simulink library "marine_hydro"  (Simulink 7.4)
settings: Solver=ode45  SolverMode=SingleTasking  StartTime=0.0  StopTime=10.0  RelTol=1e-3
undefined symbols (not defined in the file or in its folder): Hoerner, magnitude, slcm, vessel, vesselABC
libraries: simulink x60, marine_gnc x22, marine_hydro x9
(part 4 of 4)

== system marine_hydro/Hydro Library/Wave loads (U>0)/Wave loads U = U1/psi2 ==
  k : Inport  OutDataType=sfix(16)  OutScaling=2^0
  0 or 1 : Inport  Port=2  OutDataType=sfix(16)  OutScaling=2^0
  Gain1 : Gain  Gain=20  ParameterDataType=sfix(16)  ParameterScaling=2^0  OutDataType=sfix(16)  OutScaling=2^0
  Gain2 : Gain  Gain=10  ParameterDataType=sfix(16)  ParameterScaling=2^0  OutDataType=sfix(16)  OutScaling=2^0
  Product : Product  OutDataType=sfix(16)  OutScaling=2^0  RndMeth=Zero
  Sum7 : Sum  Inputs=-+|  OutDataType=sfix(16)  OutScaling=2^0
  Sum8 : Sum  Inputs=++|  OutDataType=sfix(16)  OutScaling=2^0
  const : Constant  Value=18  OutDataType=sfix(16)  OutScaling=2^0
  psi : Outport  OutDataType=sfix(16)  OutScaling=2^0
  wires:
  0 or 1/1 -> Product/2
  Sum8/1 -> psi/1
  k/1 -> Gain2/1, Sum7/1
  Gain2/1 -> Sum8/1
  Product/1 -> Sum8/2
  Gain1/1 -> Product/1
  Sum7/1 -> Gain1/1
  const/1 -> Sum7/2

== system marine_hydro/Hydro Library/Wave loads (U>0)/Wave loads U = U2/Wave loads for heading1 ==
  eta : Inport  OutDataType=sfix(16)  OutScaling=2^0
  psi : Inport  Port=2  OutDataType=sfix(16)  OutScaling=2^0
  psi_wave : Inport  Port=3  OutDataType=sfix(16)  OutScaling=2^0
  wavenum : Inport  Port=4  OutDataType=sfix(16)  OutScaling=2^0
  Omega : Inport  Port=5  OutDataType=sfix(16)  OutScaling=2^0
  Phase : Inport  Port=6  OutDataType=sfix(16)  OutScaling=2^0
  Zeta_a : Inport  Port=7  OutDataType=sfix(16)  OutScaling=2^0
  U_idx : Inport  Port=8  OutDataType=sfix(16)  OutScaling=2^0
  Clock : Clock
      settings: Decimation=10
  Position phase : marine_gnc/Models/Environmental Loads/Utilities/Position phase  SystemSampleTime=-1
  Product1 : Product  Inputs=**  OutDataType=sfix(16)  OutScaling=2^0  SaturateOnIntegerOverflow=on  OutDataTypeStr=Inherit: Same as first input
  Sum : Sum  Inputs=-++  OutDataType=sfix(16)  OutScaling=2^0  SaturateOnIntegerOverflow=on
  Sum1 : Sum  Inputs=-+|  OutDataType=sfix(16)  OutScaling=2^0
  Wave component loop : Subsystem  TreatAsAtomicUnit=on
  Width : Width  DataType=int32
  tau_WF : Outport  OutDataType=sfix(16)  OutScaling=2^0
  tau_WD : Outport  Port=2  OutDataType=sfix(16)  OutScaling=2^0
  wires:
  psi/1 -> Sum1/1  "psi"
  U_idx/1 -> Wave component loop/6(U_idx)
  Wave component loop/2(tau_WD) -> tau_WD/1
  Sum1/1 -> Wave component loop/2(Psi_r)
  Zeta_a/1 -> Wave component loop/5(Zeta_a)
  Phase/1 -> Sum/3
  Omega/1 -> Width/1, Wave component loop/3(Omega), Product1/1
  wavenum/1 -> Position phase/2
  psi_wave/1 -> Sum1/2, Position phase/1
  eta/1 -> Position phase/3
  Wave component loop/1(tau_WF) -> tau_WF/1
  Product1/1 -> Sum/2
  Clock/1 -> Product1/2
  Sum/1 -> Wave component loop/4(Phase_tot)  "Phase_tot"
  Width/1 -> Wave component loop/1(number of  iterations)
  Position phase/1 -> Sum/1

== system marine_hydro/Hydro Library/Wave loads (U>0)/Wave loads U = U2/Wave loads for heading2 ==
  eta : Inport  OutDataType=sfix(16)  OutScaling=2^0
  psi : Inport  Port=2  OutDataType=sfix(16)  OutScaling=2^0
  psi_wave : Inport  Port=3  OutDataType=sfix(16)  OutScaling=2^0
  wavenum : Inport  Port=4  OutDataType=sfix(16)  OutScaling=2^0
  Omega : Inport  Port=5  OutDataType=sfix(16)  OutScaling=2^0
  Phase : Inport  Port=6  OutDataType=sfix(16)  OutScaling=2^0
  Zeta_a : Inport  Port=7  OutDataType=sfix(16)  OutScaling=2^0
  U : Inport  Port=8  OutDataType=sfix(16)  OutScaling=2^0
  Clock : Clock
      settings: Decimation=10
  Position phase : marine_gnc/Models/Environmental Loads/Utilities/Position phase  SystemSampleTime=-1
  Product1 : Product  Inputs=**  OutDataType=sfix(16)  OutScaling=2^0  SaturateOnIntegerOverflow=on  OutDataTypeStr=Inherit: Same as first input
  Sum : Sum  Inputs=-++  OutDataType=sfix(16)  OutScaling=2^0  SaturateOnIntegerOverflow=on
  Sum1 : Sum  Inputs=-+|  OutDataType=sfix(16)  OutScaling=2^0
  Wave component loop : Subsystem  TreatAsAtomicUnit=on
  Width : Width  DataType=int32
  tau_WF : Outport  OutDataType=sfix(16)  OutScaling=2^0
  tau_WD : Outport  Port=2  OutDataType=sfix(16)  OutScaling=2^0
  wires:
  psi/1 -> Sum1/1  "psi"
  U/1 -> Wave component loop/6(U)
  Wave component loop/2(tau_WD) -> tau_WD/1
  Sum1/1 -> Wave component loop/2(Psi_r)
  Zeta_a/1 -> Wave component loop/5(Zeta_a)
  Phase/1 -> Sum/3
  Omega/1 -> Width/1, Wave component loop/3(Omega), Product1/1
  wavenum/1 -> Position phase/2
  psi_wave/1 -> Sum1/2, Position phase/1
  eta/1 -> Position phase/3
  Wave component loop/1(tau_WF) -> tau_WF/1
  Product1/1 -> Sum/2
  Clock/1 -> Product1/2
  Sum/1 -> Wave component loop/4(Phase_tot)  "Phase_tot"
  Width/1 -> Wave component loop/1(number of  iterations)
  Position phase/1 -> Sum/1

== system marine_hydro/Hydro Library/Wave loads (U>0)/Wave loads U = U2/psi1 ==
  k : Inport  OutDataType=sfix(16)  OutScaling=2^0
  0 or 1 : Inport  Port=2  OutDataType=sfix(16)  OutScaling=2^0
  Gain1 : Gain  Gain=20  ParameterDataType=sfix(16)  ParameterScaling=2^0  OutDataType=sfix(16)  OutScaling=2^0
  Gain2 : Gain  Gain=10  ParameterDataType=sfix(16)  ParameterScaling=2^0  OutDataType=sfix(16)  OutScaling=2^0
  Product : Product  OutDataType=sfix(16)  OutScaling=2^0  RndMeth=Zero
  Sum7 : Sum  Inputs=-+|  OutDataType=sfix(16)  OutScaling=2^0
  Sum8 : Sum  Inputs=++|  OutDataType=sfix(16)  OutScaling=2^0
  const : Constant  Value=18  OutDataType=sfix(16)  OutScaling=2^0
  psi : Outport  OutDataType=sfix(16)  OutScaling=2^0
  wires:
  0 or 1/1 -> Product/2
  Sum8/1 -> psi/1
  k/1 -> Gain2/1, Sum7/1
  Gain2/1 -> Sum8/1
  Product/1 -> Sum8/2
  Gain1/1 -> Product/1
  Sum7/1 -> Gain1/1
  const/1 -> Sum7/2

== system marine_hydro/Hydro Library/Wave loads (U>0)/Wave loads U = U2/psi2 ==
  k : Inport  OutDataType=sfix(16)  OutScaling=2^0
  0 or 1 : Inport  Port=2  OutDataType=sfix(16)  OutScaling=2^0
  Gain1 : Gain  Gain=20  ParameterDataType=sfix(16)  ParameterScaling=2^0  OutDataType=sfix(16)  OutScaling=2^0
  Gain2 : Gain  Gain=10  ParameterDataType=sfix(16)  ParameterScaling=2^0  OutDataType=sfix(16)  OutScaling=2^0
  Product : Product  OutDataType=sfix(16)  OutScaling=2^0  RndMeth=Zero
  Sum7 : Sum  Inputs=-+|  OutDataType=sfix(16)  OutScaling=2^0
  Sum8 : Sum  Inputs=++|  OutDataType=sfix(16)  OutScaling=2^0
  const : Constant  Value=18  OutDataType=sfix(16)  OutScaling=2^0
  psi : Outport  OutDataType=sfix(16)  OutScaling=2^0
  wires:
  0 or 1/1 -> Product/2
  Sum8/1 -> psi/1
  k/1 -> Gain2/1, Sum7/1
  Gain2/1 -> Sum8/1
  Product/1 -> Sum8/2
  Gain1/1 -> Product/1
  Sum7/1 -> Gain1/1
  const/1 -> Sum7/2

== system marine_hydro/Hydro Library/Wave loads for heading1/Wave component loop/Force RAO tables ==
  beta : Inport  OutDataType=sfix(16)  OutScaling=2^0
  w : Inport  Port=2  OutDataType=sfix(16)  OutScaling=2^0
  U : Inport  Port=3  OutDataType=sfix(16)  OutScaling=2^0
  Lookup Table (n-D) Amp1 : simulink/Lookup Tables/Lookup Table (n-D)  numDimsPopupSelect=3  bp1=ForceRAO_Freq  bp2=vessel.headings  bp3=RAO_Vel  bp4=[1:3]  bpcell={ [1:3], [1:3] }  explicitNumDims=2  searchMode=Linear Search  cacheBpFlag=on  vectorInputFlag=off  tableData=ForceRAO_Amp{1}  interpMethod=Linear  extrapMethod=None - Clip  rangeErrorMode=Warning
  Lookup Table (n-D) Amp2 : simulink/Lookup Tables/Lookup Table (n-D)  numDimsPopupSelect=3  bp1=ForceRAO_Freq  bp2=vessel.headings  bp3=RAO_Vel  bp4=[1:3]  bpcell={ [1:3], [1:3] }  explicitNumDims=2  searchMode=Linear Search  cacheBpFlag=on  vectorInputFlag=off  tableData=ForceRAO_Amp{2}  interpMethod=Linear  extrapMethod=None - Clip  rangeErrorMode=Warning
  Lookup Table (n-D) Amp3 : simulink/Lookup Tables/Lookup Table (n-D)  numDimsPopupSelect=3  bp1=ForceRAO_Freq  bp2=vessel.headings  bp3=RAO_Vel  bp4=[1:3]  bpcell={ [1:3], [1:3] }  explicitNumDims=2  searchMode=Linear Search  cacheBpFlag=on  vectorInputFlag=off  tableData=ForceRAO_Amp{3}  interpMethod=Linear  extrapMethod=None - Clip  rangeErrorMode=Warning
  Lookup Table (n-D) Amp4 : simulink/Lookup Tables/Lookup Table (n-D)  numDimsPopupSelect=3  bp1=ForceRAO_Freq  bp2=vessel.headings  bp3=RAO_Vel  bp4=[1:3]  bpcell={ [1:3], [1:3] }  explicitNumDims=2  searchMode=Linear Search  cacheBpFlag=on  vectorInputFlag=off  tableData=ForceRAO_Amp{4}  interpMethod=Linear  extrapMethod=None - Clip  rangeErrorMode=Warning
  Lookup Table (n-D) Amp5 : simulink/Lookup Tables/Lookup Table (n-D)  numDimsPopupSelect=3  bp1=ForceRAO_Freq  bp2=vessel.headings  bp3=RAO_Vel  bp4=[1:3]  bpcell={ [1:3], [1:3] }  explicitNumDims=2  searchMode=Linear Search  cacheBpFlag=on  vectorInputFlag=off  tableData=ForceRAO_Amp{5}  interpMethod=Linear  extrapMethod=None - Clip  rangeErrorMode=Warning
  Lookup Table (n-D) Amp6 : simulink/Lookup Tables/Lookup Table (n-D)  numDimsPopupSelect=3  bp1=ForceRAO_Freq  bp2=vessel.headings  bp3=RAO_Vel  bp4=[1:3]  bpcell={ [1:3], [1:3] }  explicitNumDims=2  searchMode=Linear Search  cacheBpFlag=on  vectorInputFlag=off  tableData=ForceRAO_Amp{6}  interpMethod=Linear  extrapMethod=None - Clip  rangeErrorMode=Warning
  Lookup Table (n-D) Phase : simulink/Lookup Tables/Lookup Table (n-D)  numDimsPopupSelect=3  bp1=ForceRAO_Freq  bp2=vessel.headings  bp3=RAO_Vel  bp4=[1:3]  bpcell={ [1:3], [1:3] }  explicitNumDims=2  searchMode=Linear Search  cacheBpFlag=on  vectorInputFlag=off  tableData=ForceRAO_Phase{3}  interpMethod=Linear  extrapMethod=None - Clip  rangeErrorMode=Warning
  Lookup Table (n-D) Phase1 : simulink/Lookup Tables/Lookup Table (n-D)  numDimsPopupSelect=3  bp1=ForceRAO_Freq  bp2=vessel.headings  bp3=RAO_Vel  bp4=[1:3]  bpcell={ [1:3], [1:3] }  explicitNumDims=2  searchMode=Linear Search  cacheBpFlag=on  vectorInputFlag=off  tableData=ForceRAO_Phase{1}  interpMethod=Linear  extrapMethod=None - Clip  rangeErrorMode=Warning
  Lookup Table (n-D) Phase2 : simulink/Lookup Tables/Lookup Table (n-D)  numDimsPopupSelect=3  bp1=ForceRAO_Freq  bp2=vessel.headings  bp3=RAO_Vel  bp4=[1:3]  bpcell={ [1:3], [1:3] }  explicitNumDims=2  searchMode=Linear Search  cacheBpFlag=on  vectorInputFlag=off  tableData=ForceRAO_Phase{2}  interpMethod=Linear  extrapMethod=None - Clip  rangeErrorMode=Warning
  Lookup Table (n-D) Phase4 : simulink/Lookup Tables/Lookup Table (n-D)  numDimsPopupSelect=3  bp1=ForceRAO_Freq  bp2=vessel.headings  bp3=RAO_Vel  bp4=[1:3]  bpcell={ [1:3], [1:3] }  explicitNumDims=2  searchMode=Linear Search  cacheBpFlag=on  vectorInputFlag=off  tableData=ForceRAO_Phase{4}  interpMethod=Linear  extrapMethod=None - Clip  rangeErrorMode=Warning
  Lookup Table (n-D) Phase5 : simulink/Lookup Tables/Lookup Table (n-D)  numDimsPopupSelect=3  bp1=ForceRAO_Freq  bp2=vessel.headings  bp3=RAO_Vel  bp4=[1:3]  bpcell={ [1:3], [1:3] }  explicitNumDims=2  searchMode=Linear Search  cacheBpFlag=on  vectorInputFlag=off  tableData=ForceRAO_Phase{5}  interpMethod=Linear  extrapMethod=None - Clip  rangeErrorMode=Warning
  Lookup Table (n-D) Phase6 : simulink/Lookup Tables/Lookup Table (n-D)  numDimsPopupSelect=3  bp1=ForceRAO_Freq  bp2=vessel.headings  bp3=RAO_Vel  bp4=[1:3]  bpcell={ [1:3], [1:3] }  explicitNumDims=2  searchMode=Linear Search  cacheBpFlag=on  vectorInputFlag=off  tableData=ForceRAO_Phase{6}  interpMethod=Linear  extrapMethod=None - Clip  rangeErrorMode=Warning
  Mux1 : Mux  Inputs=6
  Mux2 : Mux  Inputs=6
  amp : Outport  OutDataType=sfix(16)  OutScaling=2^0
  phase : Outport  Port=2  OutDataType=sfix(16)  OutScaling=2^0
  wires:
  Mux1/1 -> amp/1
  Mux2/1 -> phase/1
  Lookup Table (n-D) Amp6/1 -> Mux1/6
  Lookup Table (n-D) Amp2/1 -> Mux1/2
  Lookup Table (n-D) Amp5/1 -> Mux1/5
  Lookup Table (n-D) Amp3/1 -> Mux1/3
  Lookup Table (n-D) Amp1/1 -> Mux1/1
  U/1 -> Lookup Table (n-D) Phase5/3, Lookup Table (n-D) Phase6/3, Lookup Table (n-D) Phase4/3, Lookup Table (n-D) Phase/3, Lookup Table (n-D) Phase2/3, Lookup Table (n-D) Phase1/3, Lookup Table (n-D) Amp6/3, Lookup Table (n-D) Amp5/3, Lookup Table (n-D) Amp4/3, Lookup Table (n-D) Amp3/3, Lookup Table (n-D) Amp2/3, Lookup Table (n-D) Amp1/3
  Lookup Table (n-D) Amp4/1 -> Mux1/4
  Lookup Table (n-D) Phase6/1 -> Mux2/6
  Lookup Table (n-D) Phase2/1 -> Mux2/2
  Lookup Table (n-D) Phase4/1 -> Mux2/4
  beta/1 -> Lookup Table (n-D) Phase5/2, Lookup Table (n-D) Phase6/2, Lookup Table (n-D) Phase4/2, Lookup Table (n-D) Phase/2, Lookup Table (n-D) Phase2/2, Lookup Table (n-D) Phase1/2, Lookup Table (n-D) Amp6/2, Lookup Table (n-D) Amp5/2, Lookup Table (n-D) Amp4/2, Lookup Table (n-D) Amp3/2, Lookup Table (n-D) Amp2/2, Lookup Table (n-D) Amp1/2
  Lookup Table (n-D) Phase1/1 -> Mux2/1
  Lookup Table (n-D) Phase/1 -> Mux2/3
  Lookup Table (n-D) Phase5/1 -> Mux2/5
  w/1 -> Lookup Table (n-D) Phase5/1, Lookup Table (n-D) Phase6/1, Lookup Table (n-D) Phase4/1, Lookup Table (n-D) Phase/1, Lookup Table (n-D) Phase2/1, Lookup Table (n-D) Phase1/1, Lookup Table (n-D) Amp6/1, Lookup Table (n-D) Amp5/1, Lookup Table (n-D) Amp4/1, Lookup Table (n-D) Amp3/1, Lookup Table (n-D) Amp2/1, Lookup Table (n-D) Amp1/1

== system marine_hydro/Hydro Library/Wave loads for heading1/Wave component loop/WD RAO tables ==
  beta : Inport  OutDataType=sfix(16)  OutScaling=2^0
  w : Inport  Port=2  OutDataType=sfix(16)  OutScaling=2^0
  U : Inport  Port=3  OutDataType=sfix(16)  OutScaling=2^0
  Constant : Constant  Value=0  OutDataType=sfix(16)  OutScaling=2^0
  Lookup Table (n-D)  Wavedrift 1 : simulink/Lookup Tables/Lookup Table (n-D)  numDimsPopupSelect=3  bp1=WD_Freq  bp2=vessel.headings  bp3=RAO_Vel  bp4=[1:3]  bpcell={ [1:3], [1:3] }  explicitNumDims=2  searchMode=Linear Search  cacheBpFlag=on  vectorInputFlag=off  tableData=WD_Amp{1}  interpMethod=Linear  extrapMethod=None - Clip  rangeErrorMode=Warning
  Lookup Table (n-D)  Wavedrift 2 : simulink/Lookup Tables/Lookup Table (n-D)  numDimsPopupSelect=3  bp1=WD_Freq  bp2=vessel.headings  bp3=RAO_Vel  bp4=[1:3]  bpcell={ [1:3], [1:3] }  explicitNumDims=2  searchMode=Linear Search  cacheBpFlag=on  vectorInputFlag=off  tableData=WD_Amp{2}  interpMethod=Linear  extrapMethod=None - Clip  rangeErrorMode=Warning
  Lookup Table (n-D)  Wavedrift 3 : simulink/Lookup Tables/Lookup Table (n-D)  numDimsPopupSelect=3  bp1=WD_Freq  bp2=vessel.headings  bp3=RAO_Vel  bp4=[1:3]  bpcell={ [1:3], [1:3] }  explicitNumDims=2  searchMode=Linear Search  cacheBpFlag=on  vectorInputFlag=off  tableData=WD_Amp{3}  interpMethod=Linear  extrapMethod=None - Clip  rangeErrorMode=Warning
  Mux1 : Mux  Inputs=6
  amp : Outport  OutDataType=sfix(16)  OutScaling=2^0
  wires:
  Mux1/1 -> amp/1
  Lookup Table (n-D)  Wavedrift 3/1 -> Mux1/6
  Lookup Table (n-D)  Wavedrift 2/1 -> Mux1/2
  Lookup Table (n-D)  Wavedrift 1/1 -> Mux1/1
  U/1 -> Lookup Table (n-D)  Wavedrift 2/3, Lookup Table (n-D)  Wavedrift 3/3, Lookup Table (n-D)  Wavedrift 1/3
  beta/1 -> Lookup Table (n-D)  Wavedrift 2/2, Lookup Table (n-D)  Wavedrift 3/2, Lookup Table (n-D)  Wavedrift 1/2
  Constant/1 -> Mux1/3, Mux1/4, Mux1/5
  w/1 -> Lookup Table (n-D)  Wavedrift 2/1, Lookup Table (n-D)  Wavedrift 3/1, Lookup Table (n-D)  Wavedrift 1/1

== system marine_hydro/Hydro Library/Wave loads for heading1/Wave component loop/[-pi pi] to [0 2pi] ==
  note: x
  x [-pi pi] : Inport  OutDataType=sfix(16)  OutScaling=2^0
  Constant : Constant  Value=2*pi  OutDataType=sfix(16)  OutScaling=2^0
  Constant1 : Constant  Value=0  OutDataType=sfix(16)  OutScaling=2^0
  Sign : Signum
  Sum : Sum  Inputs=|++  OutDataType=sfix(16)  OutScaling=2^0  SaturateOnIntegerOverflow=on
  Switch : Switch
  0<y<2pi : Outport  OutDataType=sfix(16)  OutScaling=2^0
  wires:
  x [-pi pi]/1 -> Sign/1, Sum/2
  Switch/1 -> Sum/1
  Sum/1 -> 0<y<2pi/1
  Sign/1 -> Switch/2
  Constant/1 -> Switch/3
  Constant1/1 -> Switch/1

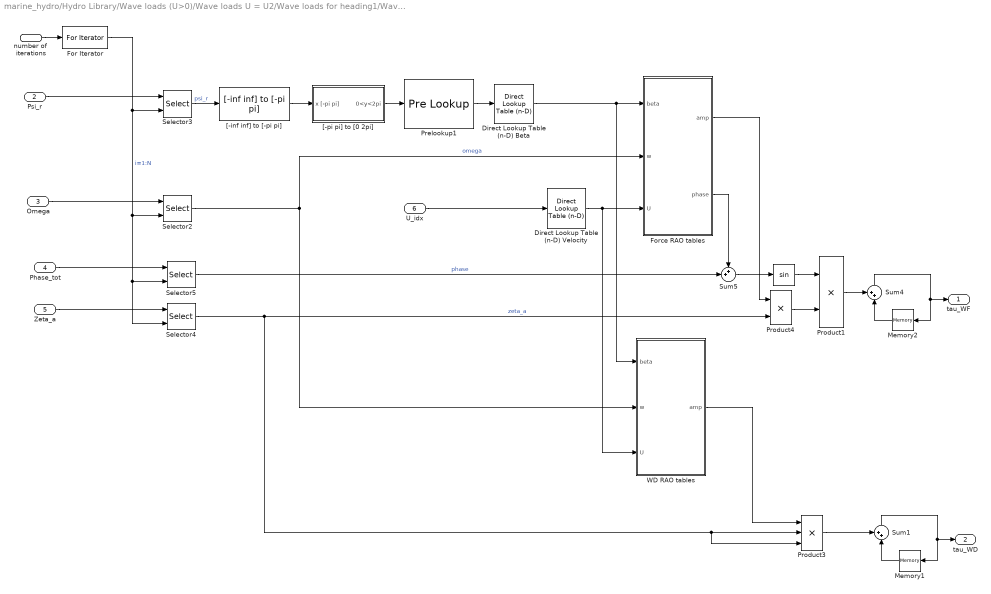
== system marine_hydro/Hydro Library/Wave loads (U>0)/Wave loads U = U2/Wave loads for heading1/Wave component loop ==
  number of  iterations : Inport  OutDataType=sfix(16)  OutScaling=2^0
  Psi_r : Inport  Port=2  OutDataType=sfix(16)  OutScaling=2^0
  Omega : Inport  Port=3  OutDataType=sfix(16)  OutScaling=2^0
  Phase_tot : Inport  Port=4  OutDataType=sfix(16)  OutScaling=2^0
  Zeta_a : Inport  Port=5  OutDataType=sfix(16)  OutScaling=2^0
  U_idx : Inport  Port=6  OutDataType=sfix(16)  OutScaling=2^0
  "                " : Trigonometry
  Direct Lookup Table (n-D) Beta : simulink/Lookup Tables/Direct Lookup Table (n-D)  maskTabDims=1  explicitNumDims=1  outDims=Element  tabIsInput=off  mxTable=vessel.headings  clipFlag=Warning  samptime=-1
  Direct Lookup Table (n-D) Velocity : simulink/Lookup Tables/Direct Lookup Table (n-D)  maskTabDims=1  explicitNumDims=1  outDims=Element  tabIsInput=off  mxTable=RAO_Vel  clipFlag=Warning  samptime=-1
  For Iterator : ForIterator  ResetStates=reset  IterationSource=external  IterationVariableDataType=double
  Force RAO tables : Subsystem  AncestorBlock=marine_gnc/Models/Environmental Loads/Utilities/RAO tables
      mask Type: RAO table lookup
      mask Description:
      | Perform 3D table lookup in 6DOF RAO amplitudes and phases, using the relative wave heading psi_r, wave frequency omega and vessel velocity vel as inputs. See documentation of the Motion RAO block or Force RAO block for details. A warning is issued if the input is outside the range spanned by the RAOs.
      | 
      | Author: Oyvind N. Smogeli and Thor I. Fossen, 2005-05-03
  Memory1 : Memory  X0=[0 0 0 0 0 0]'  InheritSampleTime=on
  Memory2 : Memory  X0=[0 0 0 0 0 0]'  InheritSampleTime=on
  Prelookup1 : PreLookup  BreakpointsData=vessel.headings  IndexSearchMethod=Evenly spaced points  BeginIndexSearchUsingPreviousIndexResult=on  OutputOnlyTheIndex=on  IndexDataType=sfix(16)  FractionDataType=sfix(16)  FractionScaling=2^0
  Product1 : Product  OutDataType=sfix(16)  OutScaling=2^0  SaturateOnIntegerOverflow=on  OutDataTypeStr=Inherit: Same as first input
  Product3 : Product  Inputs=3  OutDataType=sfix(16)  OutScaling=2^0  SaturateOnIntegerOverflow=on  OutDataTypeStr=Inherit: Same as first input
  Product4 : Product  OutDataType=sfix(16)  OutScaling=2^0  SaturateOnIntegerOverflow=on  OutDataTypeStr=Inherit: Same as first input
  Selector{2..5} (4 alike) : Selector  IndexOptions=Index vector (port)  Indices=[1 3]  OutputSizes=1
  Sum1 : Sum  Inputs=++|  OutDataType=sfix(16)  OutScaling=2^0  SaturateOnIntegerOverflow=on
  Sum4 : Sum  Inputs=++|  OutDataType=sfix(16)  OutScaling=2^0  SaturateOnIntegerOverflow=on
  Sum5 : Sum  Inputs=++|  OutDataType=sfix(16)  OutScaling=2^0  SaturateOnIntegerOverflow=on
  WD RAO tables : Subsystem  AncestorBlock=marine_gnc/Models/Environmental Loads/Utilities/RAO tables
      mask Type: RAO table lookup
      mask Description:
      | Perform 3D table lookup in 6DOF RAO amplitudes and phases, using the relative wave heading psi_r, wave frequency omega and vessel velocity vel as inputs. See documentation of the Motion RAO block or Force RAO block for details. A warning is issued if the input is outside the range spanned by the RAOs.
      | 
      | Author: Oyvind N. Smogeli and Thor I. Fossen, 2005-05-03
  "[-inf inf] to [-pi pi]" : marine_gnc/Utilities/Math Operations/[-inf inf] to [-pi pi]  SystemSampleTime=-1
  "[-pi pi] to [0 2pi]" : Subsystem
      mask Type: [-inf inf] to [-pi pi]
      mask Description: Converts an angle in rad to (-pi pi)
  tau_WF : Outport  OutDataType=sfix(16)  OutScaling=2^0
  tau_WD : Outport  Port=2  OutDataType=sfix(16)  OutScaling=2^0
  wires:
  Direct Lookup Table (n-D) Velocity/1 -> WD RAO tables/3(U), Force RAO tables/3(U)
  U_idx/1 -> Direct Lookup Table (n-D) Velocity/1
  Direct Lookup Table (n-D) Beta/1 -> WD RAO tables/1(beta), Force RAO tables/1(beta)
  Prelookup1/1 -> Direct Lookup Table (n-D) Beta/1
  "[-inf inf] to [-pi pi]"/1 -> "[-pi pi] to [0 2pi]"/1(x [-pi pi])
  For Iterator/1 -> Selector5/2, Selector4/2, Selector2/2, Selector3/2  "i=1:N"
  Selector2/1 -> WD RAO tables/2(w), Force RAO tables/2(w)  "omega"
  "[-pi pi] to [0 2pi]"/1(0<y<2pi) -> Prelookup1/1
  WD RAO tables/1(amp) -> Product3/1
  Product3/1 -> Sum1/1
  Memory1/1 -> Sum1/2
  Sum1/1 -> tau_WD/1, Memory1/1
  Product4/1 -> Product1/2
  "                "/1 -> Product1/1
  Selector3/1 -> "[-inf inf] to [-pi pi]"/1  "psi_r"
  Selector5/1 -> Sum5/2  "phase"
  Product1/1 -> Sum4/1
  Memory2/1 -> Sum4/2
  Sum4/1 -> tau_WF/1, Memory2/1
  number of  iterations/1 -> For Iterator/1
  Omega/1 -> Selector2/1
  Psi_r/1 -> Selector3/1
  Force RAO tables/1(amp) -> Product4/1
  Force RAO tables/2(phase) -> Sum5/1
  Phase_tot/1 -> Selector5/1
  Zeta_a/1 -> Selector4/1
  Sum5/1 -> "                "/1
  Selector4/1 -> Product3/3, Product3/2, Product4/2  "zeta_a"

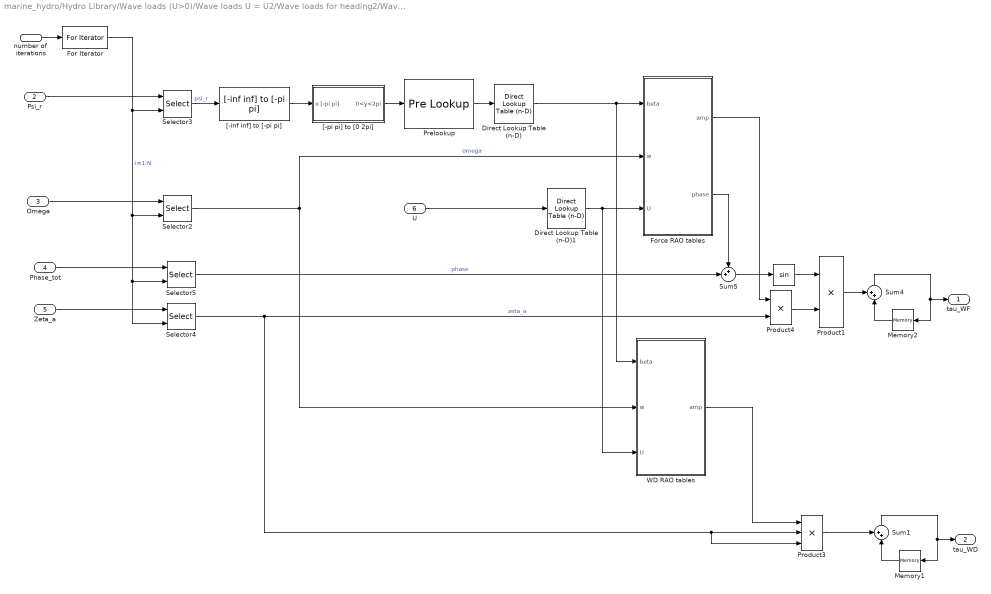
== system marine_hydro/Hydro Library/Wave loads (U>0)/Wave loads U = U2/Wave loads for heading2/Wave component loop ==
  number of  iterations : Inport  OutDataType=sfix(16)  OutScaling=2^0
  Psi_r : Inport  Port=2  OutDataType=sfix(16)  OutScaling=2^0
  Omega : Inport  Port=3  OutDataType=sfix(16)  OutScaling=2^0
  Phase_tot : Inport  Port=4  OutDataType=sfix(16)  OutScaling=2^0
  Zeta_a : Inport  Port=5  OutDataType=sfix(16)  OutScaling=2^0
  U : Inport  Port=6  OutDataType=sfix(16)  OutScaling=2^0
  "                " : Trigonometry
  Direct Lookup Table (n-D) : simulink/Lookup Tables/Direct Lookup Table (n-D)  maskTabDims=1  explicitNumDims=1  outDims=Element  tabIsInput=off  mxTable=vessel.headings  clipFlag=Warning  samptime=-1
  Direct Lookup Table (n-D)1 : simulink/Lookup Tables/Direct Lookup Table (n-D)  maskTabDims=1  explicitNumDims=1  outDims=Element  tabIsInput=off  mxTable=RAO_Vel  clipFlag=Warning  samptime=-1
  For Iterator : ForIterator  ResetStates=reset  IterationSource=external  IterationVariableDataType=double
  Force RAO tables : Subsystem  AncestorBlock=marine_gnc/Models/Environmental Loads/Utilities/RAO tables
      mask Type: RAO table lookup
      mask Description:
      | Perform 3D table lookup in 6DOF RAO amplitudes and phases, using the relative wave heading psi_r, wave frequency omega and vessel velocity vel as inputs. See documentation of the Motion RAO block or Force RAO block for details. A warning is issued if the input is outside the range spanned by the RAOs.
      | 
      | Copyright (C) NTNU 2005
      | 
      | Author: Oyvind N. Smogeli, 2005-05-03
  Memory1 : Memory  X0=[0 0 0 0 0 0]'  InheritSampleTime=on
  Memory2 : Memory  X0=[0 0 0 0 0 0]'  InheritSampleTime=on
  Prelookup : PreLookup  BreakpointsData=vessel.headings  IndexSearchMethod=Evenly spaced points  BeginIndexSearchUsingPreviousIndexResult=on  OutputOnlyTheIndex=on  IndexDataType=sfix(16)  FractionDataType=sfix(16)  FractionScaling=2^0
  Product1 : Product  OutDataType=sfix(16)  OutScaling=2^0  SaturateOnIntegerOverflow=on  OutDataTypeStr=Inherit: Same as first input
  Product3 : Product  Inputs=3  OutDataType=sfix(16)  OutScaling=2^0  SaturateOnIntegerOverflow=on  OutDataTypeStr=Inherit: Same as first input
  Product4 : Product  OutDataType=sfix(16)  OutScaling=2^0  SaturateOnIntegerOverflow=on  OutDataTypeStr=Inherit: Same as first input
  Selector{2..5} (4 alike) : Selector  IndexOptions=Index vector (port)  Indices=[1 3]  OutputSizes=1
  Sum1 : Sum  Inputs=++|  OutDataType=sfix(16)  OutScaling=2^0  SaturateOnIntegerOverflow=on
  Sum4 : Sum  Inputs=++|  OutDataType=sfix(16)  OutScaling=2^0  SaturateOnIntegerOverflow=on
  Sum5 : Sum  Inputs=++|  OutDataType=sfix(16)  OutScaling=2^0  SaturateOnIntegerOverflow=on
  WD RAO tables : Subsystem  AncestorBlock=marine_gnc/Models/Environmental Loads/Utilities/RAO tables
      mask Type: RAO table lookup
      mask Description:
      | Perform 3D table lookup in 6DOF RAO amplitudes and phases, using the relative wave heading psi_r, wave frequency omega and vessel velocity vel as inputs. See documentation of the Motion RAO block or Force RAO block for details. A warning is issued if the input is outside the range spanned by the RAOs.
      | 
      | Copyright (C) NTNU 2005
      | 
      | Author: Oyvind N. Smogeli, 2005-05-03
  "[-inf inf] to [-pi pi]" : marine_gnc/Utilities/Math Operations/[-inf inf] to [-pi pi]  SystemSampleTime=-1
  "[-pi pi] to [0 2pi]" : Subsystem
      mask Type: [-inf inf] to [-pi pi]
      mask Description: Converts an angle in rad to (-pi pi)
  tau_WF : Outport  OutDataType=sfix(16)  OutScaling=2^0
  tau_WD : Outport  Port=2  OutDataType=sfix(16)  OutScaling=2^0
  wires:
  Direct Lookup Table (n-D)1/1 -> WD RAO tables/3(U), Force RAO tables/3(U)
  Direct Lookup Table (n-D)/1 -> WD RAO tables/1(beta), Force RAO tables/1(beta)
  Prelookup/1 -> Direct Lookup Table (n-D)/1
  "[-inf inf] to [-pi pi]"/1 -> "[-pi pi] to [0 2pi]"/1(x [-pi pi])
  For Iterator/1 -> Selector5/2, Selector4/2, Selector2/2, Selector3/2  "i=1:N"
  Selector2/1 -> WD RAO tables/2(w), Force RAO tables/2(w)  "omega"
  "[-pi pi] to [0 2pi]"/1(0<y<2pi) -> Prelookup/1
  WD RAO tables/1(amp) -> Product3/1
  Product3/1 -> Sum1/1
  Memory1/1 -> Sum1/2
  Sum1/1 -> tau_WD/1, Memory1/1
  Product4/1 -> Product1/2
  "                "/1 -> Product1/1
  Selector3/1 -> "[-inf inf] to [-pi pi]"/1  "psi_r"
  Selector5/1 -> Sum5/2  "phase"
  Product1/1 -> Sum4/1
  Memory2/1 -> Sum4/2
  Sum4/1 -> tau_WF/1, Memory2/1
  number of  iterations/1 -> For Iterator/1
  Omega/1 -> Selector2/1
  Psi_r/1 -> Selector3/1
  U/1 -> Direct Lookup Table (n-D)1/1
  Force RAO tables/1(amp) -> Product4/1
  Force RAO tables/2(phase) -> Sum5/1
  Phase_tot/1 -> Selector5/1
  Zeta_a/1 -> Selector4/1
  Sum5/1 -> "                "/1
  Selector4/1 -> Product3/3, Product3/2, Product4/2  "zeta_a"

== system marine_hydro/Hydro Library/Wave loads (U>0)/Wave loads U = U2/Wave loads for heading1/Wave component loop/Force RAO tables ==
  beta : Inport  OutDataType=sfix(16)  OutScaling=2^0
  w : Inport  Port=2  OutDataType=sfix(16)  OutScaling=2^0
  U : Inport  Port=3  OutDataType=sfix(16)  OutScaling=2^0
  Lookup Table (n-D) Amp1 : simulink/Lookup Tables/Lookup Table (n-D)  numDimsPopupSelect=3  bp1=ForceRAO_Freq  bp2=vessel.headings  bp3=RAO_Vel  bp4=[1:3]  bpcell={ [1:3], [1:3] }  explicitNumDims=2  searchMode=Linear Search  cacheBpFlag=on  vectorInputFlag=off  tableData=ForceRAO_Amp{1}  interpMethod=Linear  extrapMethod=None - Clip  rangeErrorMode=Warning
  Lookup Table (n-D) Amp2 : simulink/Lookup Tables/Lookup Table (n-D)  numDimsPopupSelect=3  bp1=ForceRAO_Freq  bp2=vessel.headings  bp3=RAO_Vel  bp4=[1:3]  bpcell={ [1:3], [1:3] }  explicitNumDims=2  searchMode=Linear Search  cacheBpFlag=on  vectorInputFlag=off  tableData=ForceRAO_Amp{2}  interpMethod=Linear  extrapMethod=None - Clip  rangeErrorMode=Warning
  Lookup Table (n-D) Amp3 : simulink/Lookup Tables/Lookup Table (n-D)  numDimsPopupSelect=3  bp1=ForceRAO_Freq  bp2=vessel.headings  bp3=RAO_Vel  bp4=[1:3]  bpcell={ [1:3], [1:3] }  explicitNumDims=2  searchMode=Linear Search  cacheBpFlag=on  vectorInputFlag=off  tableData=ForceRAO_Amp{3}  interpMethod=Linear  extrapMethod=None - Clip  rangeErrorMode=Warning
  Lookup Table (n-D) Amp4 : simulink/Lookup Tables/Lookup Table (n-D)  numDimsPopupSelect=3  bp1=ForceRAO_Freq  bp2=vessel.headings  bp3=RAO_Vel  bp4=[1:3]  bpcell={ [1:3], [1:3] }  explicitNumDims=2  searchMode=Linear Search  cacheBpFlag=on  vectorInputFlag=off  tableData=ForceRAO_Amp{4}  interpMethod=Linear  extrapMethod=None - Clip  rangeErrorMode=Warning
  Lookup Table (n-D) Amp5 : simulink/Lookup Tables/Lookup Table (n-D)  numDimsPopupSelect=3  bp1=ForceRAO_Freq  bp2=vessel.headings  bp3=RAO_Vel  bp4=[1:3]  bpcell={ [1:3], [1:3] }  explicitNumDims=2  searchMode=Linear Search  cacheBpFlag=on  vectorInputFlag=off  tableData=ForceRAO_Amp{5}  interpMethod=Linear  extrapMethod=None - Clip  rangeErrorMode=Warning
  Lookup Table (n-D) Amp6 : simulink/Lookup Tables/Lookup Table (n-D)  numDimsPopupSelect=3  bp1=ForceRAO_Freq  bp2=vessel.headings  bp3=RAO_Vel  bp4=[1:3]  bpcell={ [1:3], [1:3] }  explicitNumDims=2  searchMode=Linear Search  cacheBpFlag=on  vectorInputFlag=off  tableData=ForceRAO_Amp{6}  interpMethod=Linear  extrapMethod=None - Clip  rangeErrorMode=Warning
  Lookup Table (n-D) Phase : simulink/Lookup Tables/Lookup Table (n-D)  numDimsPopupSelect=3  bp1=ForceRAO_Freq  bp2=vessel.headings  bp3=RAO_Vel  bp4=[1:3]  bpcell={ [1:3], [1:3] }  explicitNumDims=2  searchMode=Linear Search  cacheBpFlag=on  vectorInputFlag=off  tableData=ForceRAO_Phase{3}  interpMethod=Linear  extrapMethod=None - Clip  rangeErrorMode=Warning
  Lookup Table (n-D) Phase1 : simulink/Lookup Tables/Lookup Table (n-D)  numDimsPopupSelect=3  bp1=ForceRAO_Freq  bp2=vessel.headings  bp3=RAO_Vel  bp4=[1:3]  bpcell={ [1:3], [1:3] }  explicitNumDims=2  searchMode=Linear Search  cacheBpFlag=on  vectorInputFlag=off  tableData=ForceRAO_Phase{1}  interpMethod=Linear  extrapMethod=None - Clip  rangeErrorMode=Warning
  Lookup Table (n-D) Phase2 : simulink/Lookup Tables/Lookup Table (n-D)  numDimsPopupSelect=3  bp1=ForceRAO_Freq  bp2=vessel.headings  bp3=RAO_Vel  bp4=[1:3]  bpcell={ [1:3], [1:3] }  explicitNumDims=2  searchMode=Linear Search  cacheBpFlag=on  vectorInputFlag=off  tableData=ForceRAO_Phase{2}  interpMethod=Linear  extrapMethod=None - Clip  rangeErrorMode=Warning
  Lookup Table (n-D) Phase4 : simulink/Lookup Tables/Lookup Table (n-D)  numDimsPopupSelect=3  bp1=ForceRAO_Freq  bp2=vessel.headings  bp3=RAO_Vel  bp4=[1:3]  bpcell={ [1:3], [1:3] }  explicitNumDims=2  searchMode=Linear Search  cacheBpFlag=on  vectorInputFlag=off  tableData=ForceRAO_Phase{4}  interpMethod=Linear  extrapMethod=None - Clip  rangeErrorMode=Warning
  Lookup Table (n-D) Phase5 : simulink/Lookup Tables/Lookup Table (n-D)  numDimsPopupSelect=3  bp1=ForceRAO_Freq  bp2=vessel.headings  bp3=RAO_Vel  bp4=[1:3]  bpcell={ [1:3], [1:3] }  explicitNumDims=2  searchMode=Linear Search  cacheBpFlag=on  vectorInputFlag=off  tableData=ForceRAO_Phase{5}  interpMethod=Linear  extrapMethod=None - Clip  rangeErrorMode=Warning
  Lookup Table (n-D) Phase6 : simulink/Lookup Tables/Lookup Table (n-D)  numDimsPopupSelect=3  bp1=ForceRAO_Freq  bp2=vessel.headings  bp3=RAO_Vel  bp4=[1:3]  bpcell={ [1:3], [1:3] }  explicitNumDims=2  searchMode=Linear Search  cacheBpFlag=on  vectorInputFlag=off  tableData=ForceRAO_Phase{6}  interpMethod=Linear  extrapMethod=None - Clip  rangeErrorMode=Warning
  Mux1 : Mux  Inputs=6
  Mux2 : Mux  Inputs=6
  amp : Outport  OutDataType=sfix(16)  OutScaling=2^0
  phase : Outport  Port=2  OutDataType=sfix(16)  OutScaling=2^0
  wires:
  w/1 -> Lookup Table (n-D) Amp1/1, Lookup Table (n-D) Amp2/1, Lookup Table (n-D) Amp3/1, Lookup Table (n-D) Amp4/1, Lookup Table (n-D) Amp5/1, Lookup Table (n-D) Amp6/1, Lookup Table (n-D) Phase1/1, Lookup Table (n-D) Phase2/1, Lookup Table (n-D) Phase/1, Lookup Table (n-D) Phase4/1, Lookup Table (n-D) Phase6/1, Lookup Table (n-D) Phase5/1
  Lookup Table (n-D) Phase5/1 -> Mux2/5
  Lookup Table (n-D) Phase/1 -> Mux2/3
  Lookup Table (n-D) Phase1/1 -> Mux2/1
  beta/1 -> Lookup Table (n-D) Amp1/2, Lookup Table (n-D) Amp2/2, Lookup Table (n-D) Amp3/2, Lookup Table (n-D) Amp4/2, Lookup Table (n-D) Amp5/2, Lookup Table (n-D) Amp6/2, Lookup Table (n-D) Phase1/2, Lookup Table (n-D) Phase2/2, Lookup Table (n-D) Phase/2, Lookup Table (n-D) Phase4/2, Lookup Table (n-D) Phase6/2, Lookup Table (n-D) Phase5/2
  Lookup Table (n-D) Phase4/1 -> Mux2/4
  Lookup Table (n-D) Phase2/1 -> Mux2/2
  Lookup Table (n-D) Phase6/1 -> Mux2/6
  Lookup Table (n-D) Amp4/1 -> Mux1/4
  U/1 -> Lookup Table (n-D) Amp1/3, Lookup Table (n-D) Amp2/3, Lookup Table (n-D) Amp3/3, Lookup Table (n-D) Amp4/3, Lookup Table (n-D) Amp5/3, Lookup Table (n-D) Amp6/3, Lookup Table (n-D) Phase1/3, Lookup Table (n-D) Phase2/3, Lookup Table (n-D) Phase/3, Lookup Table (n-D) Phase4/3, Lookup Table (n-D) Phase6/3, Lookup Table (n-D) Phase5/3
  Lookup Table (n-D) Amp1/1 -> Mux1/1
  Lookup Table (n-D) Amp3/1 -> Mux1/3
  Lookup Table (n-D) Amp5/1 -> Mux1/5
  Lookup Table (n-D) Amp2/1 -> Mux1/2
  Lookup Table (n-D) Amp6/1 -> Mux1/6
  Mux2/1 -> phase/1
  Mux1/1 -> amp/1

== system marine_hydro/Hydro Library/Wave loads (U>0)/Wave loads U = U2/Wave loads for heading1/Wave component loop/WD RAO tables ==
  beta : Inport  OutDataType=sfix(16)  OutScaling=2^0
  w : Inport  Port=2  OutDataType=sfix(16)  OutScaling=2^0
  U : Inport  Port=3  OutDataType=sfix(16)  OutScaling=2^0
  Constant : Constant  Value=0  OutDataType=sfix(16)  OutScaling=2^0
  Lookup Table (n-D)  Wavedrift 1 : simulink/Lookup Tables/Lookup Table (n-D)  numDimsPopupSelect=3  bp1=WD_Freq  bp2=vessel.headings  bp3=RAO_Vel  bp4=[1:3]  bpcell={ [1:3], [1:3] }  explicitNumDims=2  searchMode=Linear Search  cacheBpFlag=on  vectorInputFlag=off  tableData=WD_Amp{1}  interpMethod=Linear  extrapMethod=None - Clip  rangeErrorMode=Warning
  Lookup Table (n-D)  Wavedrift 2 : simulink/Lookup Tables/Lookup Table (n-D)  numDimsPopupSelect=3  bp1=WD_Freq  bp2=vessel.headings  bp3=RAO_Vel  bp4=[1:3]  bpcell={ [1:3], [1:3] }  explicitNumDims=2  searchMode=Linear Search  cacheBpFlag=on  vectorInputFlag=off  tableData=WD_Amp{2}  interpMethod=Linear  extrapMethod=None - Clip  rangeErrorMode=Warning
  Lookup Table (n-D)  Wavedrift 3 : simulink/Lookup Tables/Lookup Table (n-D)  numDimsPopupSelect=3  bp1=WD_Freq  bp2=vessel.headings  bp3=RAO_Vel  bp4=[1:3]  bpcell={ [1:3], [1:3] }  explicitNumDims=2  searchMode=Linear Search  cacheBpFlag=on  vectorInputFlag=off  tableData=WD_Amp{3}  interpMethod=Linear  extrapMethod=None - Clip  rangeErrorMode=Warning
  Mux1 : Mux  Inputs=6
  amp : Outport  OutDataType=sfix(16)  OutScaling=2^0
  wires:
  w/1 -> Lookup Table (n-D)  Wavedrift 1/1, Lookup Table (n-D)  Wavedrift 3/1, Lookup Table (n-D)  Wavedrift 2/1
  Constant/1 -> Mux1/5, Mux1/4, Mux1/3
  beta/1 -> Lookup Table (n-D)  Wavedrift 1/2, Lookup Table (n-D)  Wavedrift 3/2, Lookup Table (n-D)  Wavedrift 2/2
  U/1 -> Lookup Table (n-D)  Wavedrift 1/3, Lookup Table (n-D)  Wavedrift 3/3, Lookup Table (n-D)  Wavedrift 2/3
  Lookup Table (n-D)  Wavedrift 1/1 -> Mux1/1
  Lookup Table (n-D)  Wavedrift 2/1 -> Mux1/2
  Lookup Table (n-D)  Wavedrift 3/1 -> Mux1/6
  Mux1/1 -> amp/1

== system marine_hydro/Hydro Library/Wave loads (U>0)/Wave loads U = U2/Wave loads for heading1/Wave component loop/[-pi pi] to [0 2pi] ==
  note: x
  x [-pi pi] : Inport  OutDataType=sfix(16)  OutScaling=2^0
  Constant : Constant  Value=2*pi  OutDataType=sfix(16)  OutScaling=2^0
  Constant1 : Constant  Value=0  OutDataType=sfix(16)  OutScaling=2^0
  Sign : Signum
  Sum : Sum  Inputs=|++  OutDataType=sfix(16)  OutScaling=2^0  SaturateOnIntegerOverflow=on
  Switch : Switch
  0<y<2pi : Outport  OutDataType=sfix(16)  OutScaling=2^0
  wires:
  Constant1/1 -> Switch/1
  Constant/1 -> Switch/3
  Sign/1 -> Switch/2
  Sum/1 -> 0<y<2pi/1
  Switch/1 -> Sum/1
  x [-pi pi]/1 -> Sum/2, Sign/1

== system marine_hydro/Hydro Library/Wave loads (U>0)/Wave loads U = U2/Wave loads for heading2/Wave component loop/Force RAO tables ==
  beta : Inport  OutDataType=sfix(16)  OutScaling=2^0
  w : Inport  Port=2  OutDataType=sfix(16)  OutScaling=2^0
  U : Inport  Port=3  OutDataType=sfix(16)  OutScaling=2^0
  Lookup Table (n-D) Amp1 : simulink/Lookup Tables/Lookup Table (n-D)  numDimsPopupSelect=3  bp1=ForceRAO_Freq  bp2=vessel.headings  bp3=RAO_Vel  bp4=[1:3]  bpcell={ [1:3], [1:3] }  explicitNumDims=2  searchMode=Linear Search  cacheBpFlag=on  vectorInputFlag=off  tableData=ForceRAO_Amp{1}  interpMethod=Linear  extrapMethod=None - Clip  rangeErrorMode=Warning
  Lookup Table (n-D) Amp2 : simulink/Lookup Tables/Lookup Table (n-D)  numDimsPopupSelect=3  bp1=ForceRAO_Freq  bp2=vessel.headings  bp3=RAO_Vel  bp4=[1:3]  bpcell={ [1:3], [1:3] }  explicitNumDims=2  searchMode=Linear Search  cacheBpFlag=on  vectorInputFlag=off  tableData=ForceRAO_Amp{2}  interpMethod=Linear  extrapMethod=None - Clip  rangeErrorMode=Warning
  Lookup Table (n-D) Amp3 : simulink/Lookup Tables/Lookup Table (n-D)  numDimsPopupSelect=3  bp1=ForceRAO_Freq  bp2=vessel.headings  bp3=RAO_Vel  bp4=[1:3]  bpcell={ [1:3], [1:3] }  explicitNumDims=2  searchMode=Linear Search  cacheBpFlag=on  vectorInputFlag=off  tableData=ForceRAO_Amp{3}  interpMethod=Linear  extrapMethod=None - Clip  rangeErrorMode=Warning
  Lookup Table (n-D) Amp4 : simulink/Lookup Tables/Lookup Table (n-D)  numDimsPopupSelect=3  bp1=ForceRAO_Freq  bp2=vessel.headings  bp3=RAO_Vel  bp4=[1:3]  bpcell={ [1:3], [1:3] }  explicitNumDims=2  searchMode=Linear Search  cacheBpFlag=on  vectorInputFlag=off  tableData=ForceRAO_Amp{4}  interpMethod=Linear  extrapMethod=None - Clip  rangeErrorMode=Warning
  Lookup Table (n-D) Amp5 : simulink/Lookup Tables/Lookup Table (n-D)  numDimsPopupSelect=3  bp1=ForceRAO_Freq  bp2=vessel.headings  bp3=RAO_Vel  bp4=[1:3]  bpcell={ [1:3], [1:3] }  explicitNumDims=2  searchMode=Linear Search  cacheBpFlag=on  vectorInputFlag=off  tableData=ForceRAO_Amp{5}  interpMethod=Linear  extrapMethod=None - Clip  rangeErrorMode=Warning
  Lookup Table (n-D) Amp6 : simulink/Lookup Tables/Lookup Table (n-D)  numDimsPopupSelect=3  bp1=ForceRAO_Freq  bp2=vessel.headings  bp3=RAO_Vel  bp4=[1:3]  bpcell={ [1:3], [1:3] }  explicitNumDims=2  searchMode=Linear Search  cacheBpFlag=on  vectorInputFlag=off  tableData=ForceRAO_Amp{6}  interpMethod=Linear  extrapMethod=None - Clip  rangeErrorMode=Warning
  Lookup Table (n-D) Phase : simulink/Lookup Tables/Lookup Table (n-D)  numDimsPopupSelect=3  bp1=ForceRAO_Freq  bp2=vessel.headings  bp3=RAO_Vel  bp4=[1:3]  bpcell={ [1:3], [1:3] }  explicitNumDims=2  searchMode=Linear Search  cacheBpFlag=on  vectorInputFlag=off  tableData=ForceRAO_Phase{3}  interpMethod=Linear  extrapMethod=None - Clip  rangeErrorMode=Warning
  Lookup Table (n-D) Phase1 : simulink/Lookup Tables/Lookup Table (n-D)  numDimsPopupSelect=3  bp1=ForceRAO_Freq  bp2=vessel.headings  bp3=RAO_Vel  bp4=[1:3]  bpcell={ [1:3], [1:3] }  explicitNumDims=2  searchMode=Linear Search  cacheBpFlag=on  vectorInputFlag=off  tableData=ForceRAO_Phase{1}  interpMethod=Linear  extrapMethod=None - Clip  rangeErrorMode=Warning
  Lookup Table (n-D) Phase2 : simulink/Lookup Tables/Lookup Table (n-D)  numDimsPopupSelect=3  bp1=ForceRAO_Freq  bp2=vessel.headings  bp3=RAO_Vel  bp4=[1:3]  bpcell={ [1:3], [1:3] }  explicitNumDims=2  searchMode=Linear Search  cacheBpFlag=on  vectorInputFlag=off  tableData=ForceRAO_Phase{2}  interpMethod=Linear  extrapMethod=None - Clip  rangeErrorMode=Warning
  Lookup Table (n-D) Phase4 : simulink/Lookup Tables/Lookup Table (n-D)  numDimsPopupSelect=3  bp1=ForceRAO_Freq  bp2=vessel.headings  bp3=RAO_Vel  bp4=[1:3]  bpcell={ [1:3], [1:3] }  explicitNumDims=2  searchMode=Linear Search  cacheBpFlag=on  vectorInputFlag=off  tableData=ForceRAO_Phase{4}  interpMethod=Linear  extrapMethod=None - Clip  rangeErrorMode=Warning
  Lookup Table (n-D) Phase5 : simulink/Lookup Tables/Lookup Table (n-D)  numDimsPopupSelect=3  bp1=ForceRAO_Freq  bp2=vessel.headings  bp3=RAO_Vel  bp4=[1:3]  bpcell={ [1:3], [1:3] }  explicitNumDims=2  searchMode=Linear Search  cacheBpFlag=on  vectorInputFlag=off  tableData=ForceRAO_Phase{5}  interpMethod=Linear  extrapMethod=None - Clip  rangeErrorMode=Warning
  Lookup Table (n-D) Phase6 : simulink/Lookup Tables/Lookup Table (n-D)  numDimsPopupSelect=3  bp1=ForceRAO_Freq  bp2=vessel.headings  bp3=RAO_Vel  bp4=[1:3]  bpcell={ [1:3], [1:3] }  explicitNumDims=2  searchMode=Linear Search  cacheBpFlag=on  vectorInputFlag=off  tableData=ForceRAO_Phase{6}  interpMethod=Linear  extrapMethod=None - Clip  rangeErrorMode=Warning
  Mux1 : Mux  Inputs=6
  Mux2 : Mux  Inputs=6
  amp : Outport  OutDataType=sfix(16)  OutScaling=2^0
  phase : Outport  Port=2  OutDataType=sfix(16)  OutScaling=2^0
  wires:
  w/1 -> Lookup Table (n-D) Amp1/1, Lookup Table (n-D) Amp2/1, Lookup Table (n-D) Amp3/1, Lookup Table (n-D) Amp4/1, Lookup Table (n-D) Amp5/1, Lookup Table (n-D) Amp6/1, Lookup Table (n-D) Phase1/1, Lookup Table (n-D) Phase2/1, Lookup Table (n-D) Phase/1, Lookup Table (n-D) Phase4/1, Lookup Table (n-D) Phase6/1, Lookup Table (n-D) Phase5/1
  Lookup Table (n-D) Phase5/1 -> Mux2/5
  Lookup Table (n-D) Phase/1 -> Mux2/3
  Lookup Table (n-D) Phase1/1 -> Mux2/1
  beta/1 -> Lookup Table (n-D) Amp1/2, Lookup Table (n-D) Amp2/2, Lookup Table (n-D) Amp3/2, Lookup Table (n-D) Amp4/2, Lookup Table (n-D) Amp5/2, Lookup Table (n-D) Amp6/2, Lookup Table (n-D) Phase1/2, Lookup Table (n-D) Phase2/2, Lookup Table (n-D) Phase/2, Lookup Table (n-D) Phase4/2, Lookup Table (n-D) Phase6/2, Lookup Table (n-D) Phase5/2
  Lookup Table (n-D) Phase4/1 -> Mux2/4
  Lookup Table (n-D) Phase2/1 -> Mux2/2
  Lookup Table (n-D) Phase6/1 -> Mux2/6
  Lookup Table (n-D) Amp4/1 -> Mux1/4
  U/1 -> Lookup Table (n-D) Amp1/3, Lookup Table (n-D) Amp2/3, Lookup Table (n-D) Amp3/3, Lookup Table (n-D) Amp4/3, Lookup Table (n-D) Amp5/3, Lookup Table (n-D) Amp6/3, Lookup Table (n-D) Phase1/3, Lookup Table (n-D) Phase2/3, Lookup Table (n-D) Phase/3, Lookup Table (n-D) Phase4/3, Lookup Table (n-D) Phase6/3, Lookup Table (n-D) Phase5/3
  Lookup Table (n-D) Amp1/1 -> Mux1/1
  Lookup Table (n-D) Amp3/1 -> Mux1/3
  Lookup Table (n-D) Amp5/1 -> Mux1/5
  Lookup Table (n-D) Amp2/1 -> Mux1/2
  Lookup Table (n-D) Amp6/1 -> Mux1/6
  Mux2/1 -> phase/1
  Mux1/1 -> amp/1

== system marine_hydro/Hydro Library/Wave loads (U>0)/Wave loads U = U2/Wave loads for heading2/Wave component loop/WD RAO tables ==
  beta : Inport  OutDataType=sfix(16)  OutScaling=2^0
  w : Inport  Port=2  OutDataType=sfix(16)  OutScaling=2^0
  U : Inport  Port=3  OutDataType=sfix(16)  OutScaling=2^0
  Constant : Constant  Value=0  OutDataType=sfix(16)  OutScaling=2^0
  Lookup Table (n-D)  Wavedrift 1 : simulink/Lookup Tables/Lookup Table (n-D)  numDimsPopupSelect=3  bp1=WD_Freq  bp2=vessel.headings  bp3=RAO_Vel  bp4=[1:3]  bpcell={ [1:3], [1:3] }  explicitNumDims=2  searchMode=Linear Search  cacheBpFlag=on  vectorInputFlag=off  tableData=WD_Amp{1}  interpMethod=Linear  extrapMethod=None - Clip  rangeErrorMode=Warning
  Lookup Table (n-D)  Wavedrift 2 : simulink/Lookup Tables/Lookup Table (n-D)  numDimsPopupSelect=3  bp1=WD_Freq  bp2=vessel.headings  bp3=RAO_Vel  bp4=[1:3]  bpcell={ [1:3], [1:3] }  explicitNumDims=2  searchMode=Linear Search  cacheBpFlag=on  vectorInputFlag=off  tableData=WD_Amp{2}  interpMethod=Linear  extrapMethod=None - Clip  rangeErrorMode=Warning
  Lookup Table (n-D)  Wavedrift 3 : simulink/Lookup Tables/Lookup Table (n-D)  numDimsPopupSelect=3  bp1=WD_Freq  bp2=vessel.headings  bp3=RAO_Vel  bp4=[1:3]  bpcell={ [1:3], [1:3] }  explicitNumDims=2  searchMode=Linear Search  cacheBpFlag=on  vectorInputFlag=off  tableData=WD_Amp{3}  interpMethod=Linear  extrapMethod=None - Clip  rangeErrorMode=Warning
  Mux1 : Mux  Inputs=6
  amp : Outport  OutDataType=sfix(16)  OutScaling=2^0
  wires:
  w/1 -> Lookup Table (n-D)  Wavedrift 1/1, Lookup Table (n-D)  Wavedrift 3/1, Lookup Table (n-D)  Wavedrift 2/1
  Constant/1 -> Mux1/5, Mux1/4, Mux1/3
  beta/1 -> Lookup Table (n-D)  Wavedrift 1/2, Lookup Table (n-D)  Wavedrift 3/2, Lookup Table (n-D)  Wavedrift 2/2
  U/1 -> Lookup Table (n-D)  Wavedrift 1/3, Lookup Table (n-D)  Wavedrift 3/3, Lookup Table (n-D)  Wavedrift 2/3
  Lookup Table (n-D)  Wavedrift 1/1 -> Mux1/1
  Lookup Table (n-D)  Wavedrift 2/1 -> Mux1/2
  Lookup Table (n-D)  Wavedrift 3/1 -> Mux1/6
  Mux1/1 -> amp/1

== system marine_hydro/Hydro Library/Wave loads (U>0)/Wave loads U = U2/Wave loads for heading2/Wave component loop/[-pi pi] to [0 2pi] ==
  note: x
  x [-pi pi] : Inport  OutDataType=sfix(16)  OutScaling=2^0
  Constant : Constant  Value=2*pi  OutDataType=sfix(16)  OutScaling=2^0
  Constant1 : Constant  Value=0  OutDataType=sfix(16)  OutScaling=2^0
  Sign : Signum
  Sum : Sum  Inputs=|++  OutDataType=sfix(16)  OutScaling=2^0  SaturateOnIntegerOverflow=on
  Switch : Switch
  0<y<2pi : Outport  OutDataType=sfix(16)  OutScaling=2^0
  wires:
  Constant1/1 -> Switch/1
  Constant/1 -> Switch/3
  Sign/1 -> Switch/2
  Sum/1 -> 0<y<2pi/1
  Switch/1 -> Sum/1
  x [-pi pi]/1 -> Sum/2, Sign/1
